simulink model "P1"  (Simulink 7.9)
settings: Solver=ode45  StartTime=0.0  StopTime=10  RelTol=1e-3
settings Model: Creator=drewgross  LastModifiedBy=drewgross

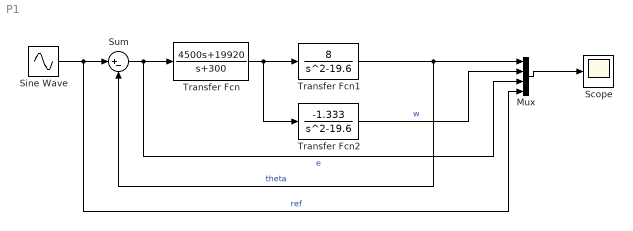
== system P1 ==
  Mux : Mux
  Scope : Scope
      settings: ShowLegends=on  TimeRange=0.01513931120593326  YMin=1.025346425692851  YMax=1.044085963171926
  Sine Wave : Sin  Frequency=0.5*2*pi  SampleTime=0
  Sum : Sum  Inputs=|+-
  Transfer Fcn : TransferFcn  Numerator=[4500 19920]  Denominator=[1 300]
  Transfer Fcn1 : TransferFcn  Numerator=[8]  Denominator=[1 0 -19.6]
  Transfer Fcn2 : TransferFcn  Numerator=[-1.333]  Denominator=[1 0 -19.6]
  wires:
  Sine Wave/1 -> Sum/1, Mux/4  "ref"
  Sum/1 -> Mux/3, Transfer Fcn/1  "e"
  Transfer Fcn/1 -> Transfer Fcn1/1, Transfer Fcn2/1
  Transfer Fcn1/1 -> Mux/1, Sum/2  "theta"
  Mux/1 -> Scope/1
  Transfer Fcn2/1 -> Mux/2  "w"
